simulink model "Cosim"  (R2020b)
settings: Solver=VariableStepAuto  StartTime=0.0  StopTime=15  RelTol=1e-3
values from neighbouring files (symbols this model uses):
  D1_Open = D1_Time + Gripper_Time    (= 4.1)    [Project_Script.m]
  D1_Time = M1_Close + Move_Time    (= 4.05)    [Project_Script.m]
  D2_Open = D2_Time + Gripper_Time    (= 10.2)    [Project_Script.m]
  D2_Time = M2_Close + Move_Time    (= 10.15)    [Project_Script.m]
  D2_Time1 = D1_Open + Move_Time    (= 6.1)    [Project_Script.m]
  D3_Time = M3_Close + Move_Time    (= 16.25)    [Project_Script.m]
  D3_Time1 = D2_Open + Move_Time    (= 12.2)    [Project_Script.m]
  Kb1 = 0.0184    [Project_Script.m]
  Km1 = 0.0184    [Project_Script.m]
  L1 = 0.000231    [Project_Script.m]
  M1_Close = M1_Time + Gripper_Time    (= 2.05)    [Project_Script.m]
  M1_Time = Move_Time    (= 2)    [Project_Script.m]
  M2_Close = M2_Time + Gripper_Time    (= 8.15)    [Project_Script.m]
  M2_Time = D2_Time1 + Move_Time    (= 8.1)    [Project_Script.m]
  M3_Close = M3_Time + Gripper_Time    (= 14.25)    [Project_Script.m]
  M3_Time = D3_Time1 + Move_Time    (= 14.2)    [Project_Script.m]
  Motor1_D1 = 0    [Project_Script.m]
  Motor1_D2 = -(360-345.73)-M1    (= -51.7)    [Project_Script.m]
  Motor1_D3 = -(360-330.2)-M1    (= -67.23)    [Project_Script.m]
  Motor1_M1 = 73.97-M1    (= 36.54)    [Project_Script.m]
  Motor1_M2 = 40.54-M1    (= 3.11)    [Project_Script.m]
  Motor1_M3 = 30.31-M1    (= -7.12)    [Project_Script.m]
  Motor2_D1 = 0    [Project_Script.m]
  Motor2_D2 = -(46.53-M2)    (= 17.05)    [Project_Script.m]
  Motor2_D3 = -(63.66-M2)    (= -0.08)    [Project_Script.m]
  Motor2_M1 = -(124.27-M2)    (= -60.69)    [Project_Script.m]
  Motor2_M2 = -(108.21-M2)    (= -44.63)    [Project_Script.m]
  Motor2_M3 = -(124.23-M2)    (= -60.65)    [Project_Script.m]
  Motor3_D1 = 0    [Project_Script.m]
  Motor3_D2 = 150.8-M3    (= 34.65)    [Project_Script.m]
  Motor3_D3 = 183.46-M3    (= 67.31)    [Project_Script.m]
  Motor3_M1 = 140.3-M3    (= 24.15)    [Project_Script.m]
  Motor3_M2 = 157.67-M3    (= 41.52)    [Project_Script.m]
  Motor3_M3 = 183.92-M3    (= 67.77)    [Project_Script.m]
  Motor4_Closed = -90    [Project_Script.m]
  Motor4_Open = 0    [Project_Script.m]
  R1 = 3.69    [Project_Script.m]
  res = 2*pi/1024    (= 0.00613592315154)    [Project_Script.m]
  Sample_Time = 10000    [Project_Script.m]
libraries: cstblocks x8
settings Model: Creator=deniz  LastModifiedBy=tnurs

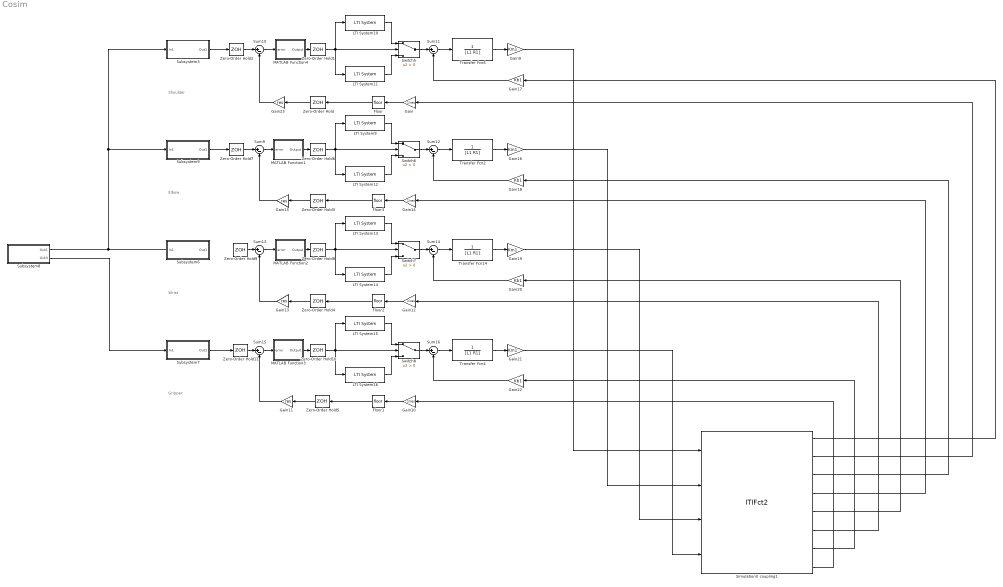
== system Cosim ==
  note: Gripper
  note: Shoulder
  note: Elbow
  note: Wrist
  Floor{,1..3} (4 alike) : Rounding
  Gain{,10,12,14} (4 alike) : Gain  Gain=1/res
  Gain{11,13,15,23} (4 alike) : Gain  Gain=res
  Gain{9,16,19,21} (4 alike) : Gain  Gain=Km1
  Gain{17..18,20,22} (4 alike) : Gain  Gain=Kb1
  LTI System{9..10,13,15} (4 alike) : cstblocks/LTI System  sys=Amp_tf_CW  IC=[]
  LTI System{11..12,14,16} (4 alike) : cstblocks/LTI System  sys=Amp_tf_CCW  IC=[]
  MATLAB Function1 : MATLAB Function  TreatAsAtomicUnit=on
  MATLAB Function2 : MATLAB Function  TreatAsAtomicUnit=on
  MATLAB Function3 : MATLAB Function  TreatAsAtomicUnit=on
  MATLAB Function4 : MATLAB Function  TreatAsAtomicUnit=on
  SimulationX coupling1 : S-Function  FunctionName=ITIFct2  Parameters=ip, port, ts, nIn, nOut  SFunctionDeploymentMode=off  EnableBusSupport=off  mask{ip='localhost', port=4097, ts=0.001, nIn=4, nOut=8}
      mask prompts: ip "Address: ip"; port "Port Number: port [-]"; ts "Communication Step Size: ts [s]"; nIn "Input Vector Dimension (to SimulationX): nIn [-]"; nOut "Output Vector Dimension (from SimulationX): nOut [-]"
      mask help: Coupling Element
  Subsystem3 : Subsystem
  Subsystem6 : Subsystem
  Subsystem7 : Subsystem
  Subsystem8 : Subsystem
  Subsystem9 : Subsystem
  Sum{9..16} (8 alike) : Sum  Inputs=|+-
  Switch{5..8} (4 alike) : Switch  Criteria=u2 > Threshold
  Transfer Fcn{2,4,6,14} (4 alike) : TransferFcn  Denominator=[L1 R1]
  Zero-Order Hold{,1..11} (12 alike) : ZeroOrderHold  SampleTime=1/Sample_Time
  wires:
  MATLAB Function3/1(Output) -> Zero-Order Hold10/1
  Sum13/1 -> MATLAB Function2/1(error)
  Zero-Order Hold1/1 -> Switch5/2, LTI System11/1, LTI System10/1
  Zero-Order Hold3/1 -> Gain15/1
  Zero-Order Hold11/1 -> Sum15/1
  Zero-Order Hold6/1 -> Switch6/2, LTI System12/1, LTI System9/1
  MATLAB Function2/1(Output) -> Zero-Order Hold8/1
  Zero-Order Hold8/1 -> Switch7/2, LTI System13/1, LTI System14/1
  Zero-Order Hold2/1 -> Sum10/1
  Zero-Order Hold5/1 -> Gain11/1
  Sum10/1 -> MATLAB Function4/1(error)
  MATLAB Function4/1(Output) -> Zero-Order Hold1/1
  Floor2/1 -> Zero-Order Hold4/1
  Sum15/1 -> MATLAB Function3/1(error)
  Floor3/1 -> Zero-Order Hold3/1
  Zero-Order Hold9/1 -> Sum13/1
  Sum9/1 -> MATLAB Function1/1(error)
  MATLAB Function1/1(Output) -> Zero-Order Hold6/1
  Gain12/1 -> Floor2/1
  Gain23/1 -> Sum10/2
  Zero-Order Hold10/1 -> Switch8/2, LTI System16/1, LTI System15/1
  Gain/1 -> Floor/1
  Zero-Order Hold/1 -> Gain23/1
  Gain14/1 -> Floor3/1
  Switch5/1 -> Sum11/1
  Floor/1 -> Zero-Order Hold/1
  Transfer Fcn6/1 -> Gain9/1
  Zero-Order Hold7/1 -> Sum9/1
  Gain17/1 -> Sum11/2
  LTI System11/1 -> Switch5/3
  Gain15/1 -> Sum9/2
  Gain11/1 -> Sum15/2
  Subsystem8/1(Out1) -> Subsystem9/1(In1), Subsystem3/1(In1)
  LTI System13/1 -> Switch7/1
  Gain13/1 -> Sum13/2
  Zero-Order Hold4/1 -> Gain13/1
  Transfer Fcn2/1 -> Gain16/1
  Sum11/1 -> Transfer Fcn6/1
  Floor1/1 -> Zero-Order Hold5/1
  LTI System9/1 -> Switch6/1
  Gain22/1 -> Sum16/2
  LTI System10/1 -> Switch5/1
  LTI System16/1 -> Switch8/3
  Sum16/1 -> Transfer Fcn4/1
  Gain18/1 -> Sum12/2
  Gain10/1 -> Floor1/1
  Transfer Fcn4/1 -> Gain21/1
  LTI System15/1 -> Switch8/1
  Sum14/1 -> Transfer Fcn14/1
  Sum12/1 -> Transfer Fcn2/1
  Switch7/1 -> Sum14/1
  Switch8/1 -> Sum16/1
  Switch6/1 -> Sum12/1
  LTI System14/1 -> Switch7/3
  Transfer Fcn14/1 -> Gain19/1
  LTI System12/1 -> Switch6/3
  Subsystem8/2(Out3) -> Subsystem7/1(In1)
  Gain20/1 -> Sum14/2
  Subsystem7/1(Out1) -> Zero-Order Hold11/1
  SimulationX coupling1/8 -> Gain10/1
  SimulationX coupling1/7 -> Gain22/1
  SimulationX coupling1/6 -> Gain12/1
  SimulationX coupling1/5 -> Gain20/1
  SimulationX coupling1/4 -> Gain14/1
  SimulationX coupling1/3 -> Gain18/1
  SimulationX coupling1/2 -> Gain/1
  SimulationX coupling1/1 -> Gain17/1
  Gain16/1 -> SimulationX coupling1/2
  Gain19/1 -> SimulationX coupling1/3
  Gain21/1 -> SimulationX coupling1/4
  Gain9/1 -> SimulationX coupling1/1
  Subsystem3/1(Out1) -> Zero-Order Hold2/1
  ? -> Zero-Order Hold9/1
  Subsystem9/1(Out1) -> Zero-Order Hold7/1

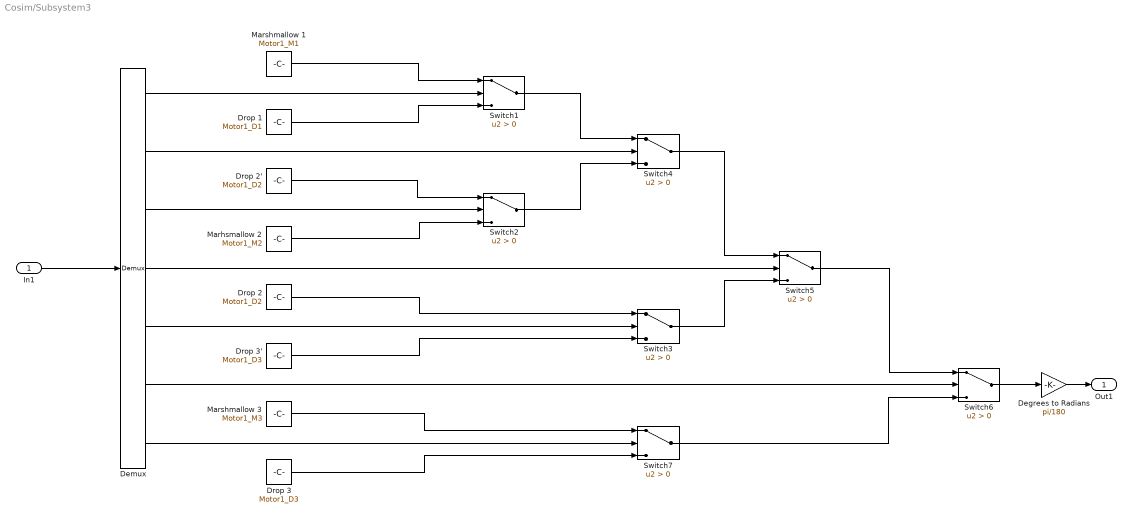
== system Cosim/Subsystem3 ==
  In1 : Inport
  Degrees to Radians : Gain  Gain=pi/180
  Demux : Demux  Outputs=7
  Drop 1 : Constant  Value=Motor1_D1
  Drop 2 : Constant  Value=Motor1_D2
  Drop 2' : Constant  Value=Motor1_D2  VectorParams1D=off
  Drop 3 : Constant  Value=Motor1_D3
  Drop 3' : Constant  Value=Motor1_D3
  Marhsmallow 2 : Constant  Value=Motor1_M2
  Marshmallow 1 : Constant  Value=Motor1_M1
  Marshmallow 3 : Constant  Value=Motor1_M3
  Switch{1..7} (7 alike) : Switch  Criteria=u2 > Threshold
  Out1 : Outport
  wires:
  Marshmallow 1/1 -> Switch1/1
  Drop 1/1 -> Switch1/3
  Drop 2'/1 -> Switch2/1
  Drop 2/1 -> Switch3/1
  Demux/3 -> Switch2/2
  Switch1/1 -> Switch4/1
  Switch2/1 -> Switch4/3
  Switch4/1 -> Switch5/1
  Switch3/1 -> Switch5/3
  Demux/2 -> Switch4/2
  Demux/4 -> Switch5/2
  Drop 3'/1 -> Switch3/3
  Demux/1 -> Switch1/2
  Degrees to Radians/1 -> Out1/1
  Demux/5 -> Switch3/2
  In1/1 -> Demux/1
  Marhsmallow 2/1 -> Switch2/3
  Demux/6 -> Switch6/2
  Switch5/1 -> Switch6/1
  Marshmallow 3/1 -> Switch7/1
  Drop 3/1 -> Switch7/3
  Switch7/1 -> Switch6/3
  Demux/7 -> Switch7/2
  Switch6/1 -> Degrees to Radians/1

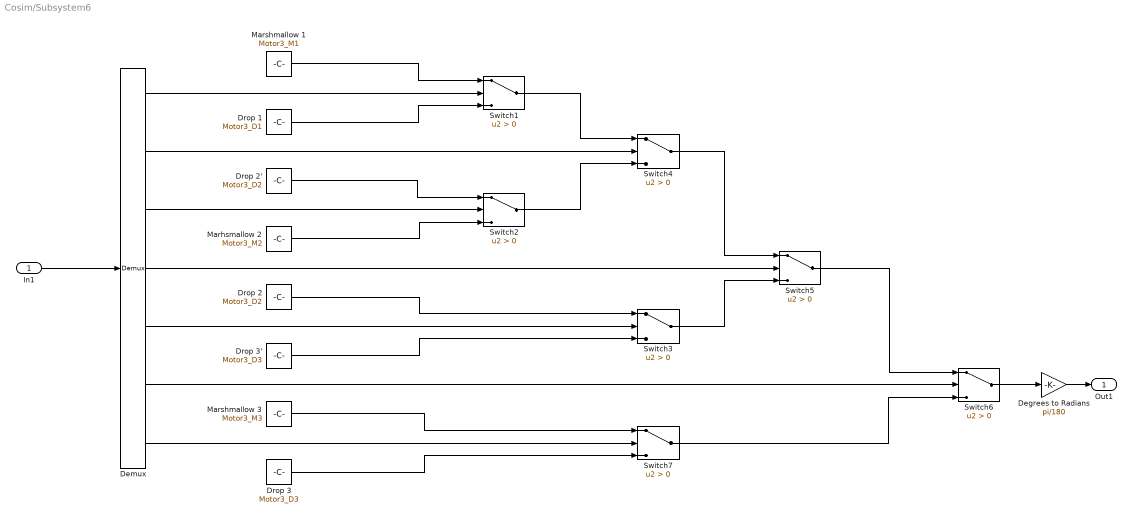
== system Cosim/Subsystem6 ==
  In1 : Inport
  Degrees to Radians : Gain  Gain=pi/180
  Demux : Demux  Outputs=7
  Drop 1 : Constant  Value=Motor3_D1
  Drop 2 : Constant  Value=Motor3_D2
  Drop 2' : Constant  Value=Motor3_D2  VectorParams1D=off
  Drop 3 : Constant  Value=Motor3_D3
  Drop 3' : Constant  Value=Motor3_D3
  Marhsmallow 2 : Constant  Value=Motor3_M2
  Marshmallow 1 : Constant  Value=Motor3_M1
  Marshmallow 3 : Constant  Value=Motor3_M3
  Switch{1..7} (7 alike) : Switch  Criteria=u2 > Threshold
  Out1 : Outport
  wires:
  Drop 3'/1 -> Switch3/3
  Demux/1 -> Switch1/2
  Demux/2 -> Switch4/2
  Marhsmallow 2/1 -> Switch2/3
  In1/1 -> Demux/1
  Drop 1/1 -> Switch1/3
  Switch5/1 -> Switch6/1
  Drop 2'/1 -> Switch2/1
  Switch3/1 -> Switch5/3
  Degrees to Radians/1 -> Out1/1
  Switch4/1 -> Switch5/1
  Switch2/1 -> Switch4/3
  Drop 2/1 -> Switch3/1
  Demux/6 -> Switch6/2
  Switch1/1 -> Switch4/1
  Marshmallow 1/1 -> Switch1/1
  Demux/4 -> Switch5/2
  Demux/7 -> Switch7/2
  Marshmallow 3/1 -> Switch7/1
  Switch6/1 -> Degrees to Radians/1
  Demux/3 -> Switch2/2
  Switch7/1 -> Switch6/3
  Drop 3/1 -> Switch7/3
  Demux/5 -> Switch3/2

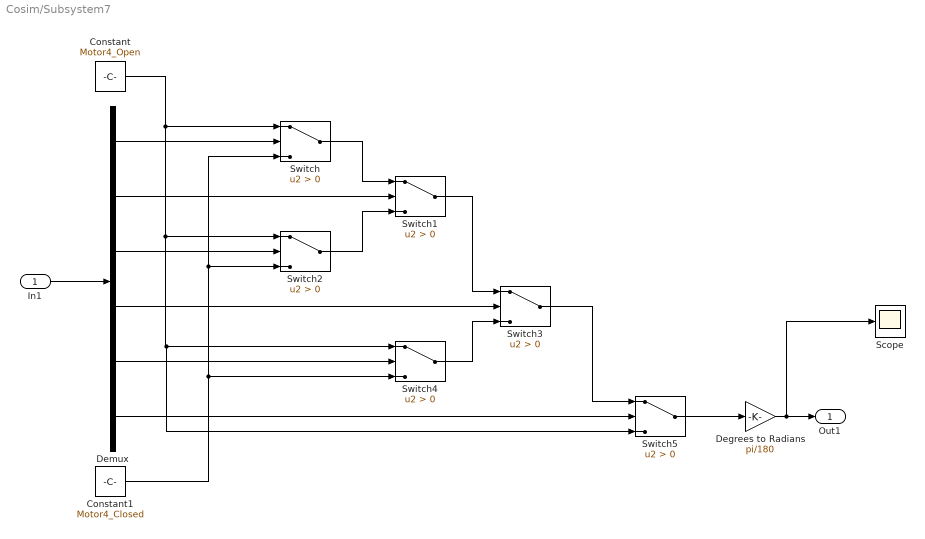
== system Cosim/Subsystem7 ==
  In1 : Inport
  Constant : Constant  Value=Motor4_Open
  Constant1 : Constant  Value=Motor4_Closed
  Degrees to Radians : Gain  Gain=pi/180
  Demux : Demux  Outputs=6
  Scope : Scope
  Switch{,1..5} (6 alike) : Switch  Criteria=u2 > Threshold
  Out1 : Outport
  wires:
  Switch5/1 -> Degrees to Radians/1
  In1/1 -> Demux/1
  Degrees to Radians/1 -> Scope/1, Out1/1
  Constant/1 -> Switch5/3, Switch4/1, Switch2/1, Switch/1
  Demux/1 -> Switch/2
  Constant1/1 -> Switch4/3, Switch2/3, Switch/3
  Demux/2 -> Switch1/2
  Switch/1 -> Switch1/1
  Switch2/1 -> Switch1/3
  Demux/3 -> Switch2/2
  Demux/4 -> Switch3/2
  Switch1/1 -> Switch3/1
  Switch4/1 -> Switch3/3
  Demux/5 -> Switch4/2
  Demux/6 -> Switch5/2
  Switch3/1 -> Switch5/1

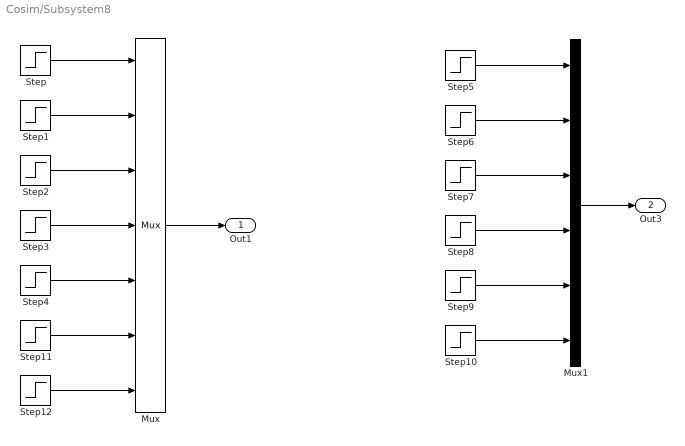
== system Cosim/Subsystem8 ==
  Mux : Mux  Inputs=7
  Mux1 : Mux  Inputs=6
  Step : Step  Time=M1_Close  Before=1  After=0  SampleTime=0
  Step1 : Step  Time=D1_Open  Before=1  After=0  SampleTime=0
  Step10 : Step  Time=D3_Time  Before=1  After=0  SampleTime=0
  Step11 : Step  Time=D3_Time1  Before=1  After=0  SampleTime=0
  Step12 : Step  Time=M3_Close  Before=1  After=0  SampleTime=0
  Step2 : Step  Time=D2_Time1  Before=1  After=0  SampleTime=0
  Step3 : Step  Time=M2_Close  Before=1  After=0  SampleTime=0
  Step4 : Step  Time=D2_Open  Before=1  After=0  SampleTime=0
  Step5 : Step  Time=M1_Time  Before=1  After=0  SampleTime=0
  Step6 : Step  Time=D1_Time  Before=1  After=0  SampleTime=0
  Step7 : Step  Time=M2_Time  Before=1  After=0  SampleTime=0
  Step8 : Step  Time=D2_Time  Before=1  After=0  SampleTime=0
  Step9 : Step  Time=M3_Time  Before=1  After=0  SampleTime=0
  Out1 : Outport
  Out3 : Outport  Port=2
  wires:
  Mux/1 -> Out1/1
  Step4/1 -> Mux/5
  Step3/1 -> Mux/4
  Step2/1 -> Mux/3
  Step1/1 -> Mux/2
  Step/1 -> Mux/1
  Step8/1 -> Mux1/4
  Step6/1 -> Mux1/2
  Step9/1 -> Mux1/5
  Mux1/1 -> Out3/1
  Step7/1 -> Mux1/3
  Step5/1 -> Mux1/1
  Step10/1 -> Mux1/6
  Step11/1 -> Mux/6
  Step12/1 -> Mux/7

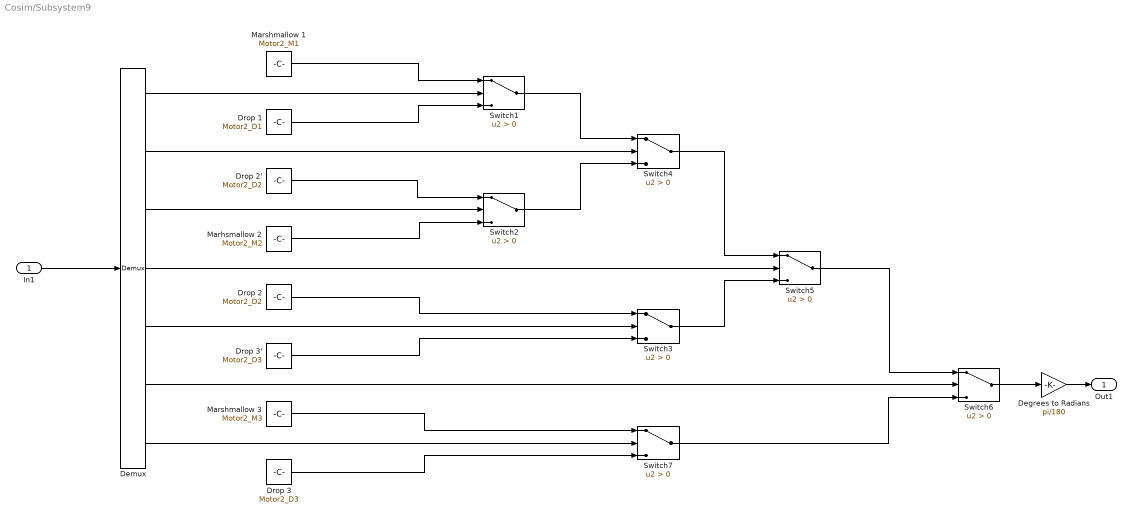
== system Cosim/Subsystem9 ==
  In1 : Inport
  Degrees to Radians : Gain  Gain=pi/180
  Demux : Demux  Outputs=7
  Drop 1 : Constant  Value=Motor2_D1
  Drop 2 : Constant  Value=Motor2_D2
  Drop 2' : Constant  Value=Motor2_D2  VectorParams1D=off
  Drop 3 : Constant  Value=Motor2_D3
  Drop 3' : Constant  Value=Motor2_D3
  Marhsmallow 2 : Constant  Value=Motor2_M2
  Marshmallow 1 : Constant  Value=Motor2_M1
  Marshmallow 3 : Constant  Value=Motor2_M3
  Switch{1..7} (7 alike) : Switch  Criteria=u2 > Threshold
  Out1 : Outport
  wires:
  Drop 3'/1 -> Switch3/3
  Demux/1 -> Switch1/2
  Demux/2 -> Switch4/2
  Marhsmallow 2/1 -> Switch2/3
  In1/1 -> Demux/1
  Drop 1/1 -> Switch1/3
  Switch5/1 -> Switch6/1
  Drop 2'/1 -> Switch2/1
  Switch3/1 -> Switch5/3
  Degrees to Radians/1 -> Out1/1
  Switch4/1 -> Switch5/1
  Switch2/1 -> Switch4/3
  Drop 2/1 -> Switch3/1
  Demux/6 -> Switch6/2
  Switch1/1 -> Switch4/1
  Marshmallow 1/1 -> Switch1/1
  Demux/4 -> Switch5/2
  Demux/7 -> Switch7/2
  Marshmallow 3/1 -> Switch7/1
  Switch6/1 -> Degrees to Radians/1
  Demux/3 -> Switch2/2
  Switch7/1 -> Switch6/3
  Drop 3/1 -> Switch7/3
  Demux/5 -> Switch3/2

== matlab function Cosim/MATLAB Function2 ==
  settings: sampleTime=1/10000
  data: error input; Output output
function Output = PID(error)

persistent ept              %holds the exponentials
persistent results          %holds reccorded derivatives
persistent previous_error   %holds input from last execution for derivative calc
persistent integral         %holds the total integral
CF = 10000;                 %ISR frequency
delta_t = 1/CF;             %Will change according to CF, sampling time
size = 8;                   %can change between 5-10
n = 4;                      %Decaying until n*tau, can be 4 or 5
pole = n*CF/size;
P_gain = 0.2616;
D_gain = 0.0432;
%I_gain = 13.390;
I_gain = 0.01;

%initialize vectors and variables
if isempty(results)
    results = zeros(1,size);
    ept = zeros(1,size);
    sum = 0;
    integral = 0;
    previous_error = 0;
    
    %calculate scale factor for derivative
    for i = 1:size
        sum = sum + pole*exp(-pole*i*delta_t);
    end
    Scale_Factor = 1/(sum);
    
    %properly create ept
    for i = 1:size
        ept(i) = Scale_Factor*pole*exp(-pole*i*delta_t);
    end
end

%Calculating the D(Derivative) of PID
results(2:size)=results(1:size-1);
results(1)=(error - previous_error)/delta_t;
previous_error = error;
derivative = dot(results,ept);

%Calculating the I(Integral) of PID
integral = integral + (error + previous_error)/2*delta_t;

%Calculating the P(Proportional) of PID
proportional = error*P_gain;

Output = proportional + I_gain*integral + D_gain*derivative;

== matlab function Cosim/MATLAB Function3 ==
  settings: sampleTime=1/10000
  data: error input; Output output
function Output = PID(error)

persistent ept              %holds the exponentials
persistent results          %holds reccorded derivatives
persistent previous_error   %holds input from last execution for derivative calc
persistent integral         %holds the total integral
CF = 10000;                 %ISR frequency
delta_t = 1/CF;             %Will change according to CF, sampling time
size = 8;                   %can change between 5-10
n = 4;                      %Decaying until n*tau, can be 4 or 5
pole = n*CF/size;
P_gain = 0.2616;
D_gain = 0.0432;
I_gain = 0.01;
%I_gain = 13.390;

%initialize vectors and variables
if isempty(results)
    results = zeros(1,size);
    ept = zeros(1,size);
    sum = 0;
    integral = 0;
    previous_error = 0;
    
    %calculate scale factor for derivative
    for i = 1:size
        sum = sum + pole*exp(-pole*i*delta_t);
    end
    Scale_Factor = 1/(sum);
    
    %properly create ept
    for i = 1:size
        ept(i) = Scale_Factor*pole*exp(-pole*i*delta_t);
    end
end

%Calculating the D(Derivative) of PID
results(2:size)=results(1:size-1);
results(1)=(error - previous_error)/delta_t;
previous_error = error;
derivative = dot(results,ept);

%Calculating the I(Integral) of PID
integral = integral + (error + previous_error)/2*delta_t;

%Calculating the P(Proportional) of PID
proportional = error*P_gain;

%Output = proportional;
Output = proportional + I_gain*integral + D_gain*derivative;

== matlab function Cosim/MATLAB Function4 ==
  settings: sampleTime=1/10000
  data: error input; Output output
function Output = PID(error)

persistent ept              %holds the exponentials
persistent results          %holds reccorded derivatives
persistent previous_error   %holds input from last execution for derivative calc
persistent integral         %holds the total integral
CF = 10000;                 %ISR frequency
delta_t = 1/CF;             %Will change according to CF, sampling time
size = 8;                   %can change between 5-10
n = 4;                      %Decaying until n*tau, can be 4 or 5
pole = n*CF/size;
P_gain = 0.2616;
%P_gain = 0.2616;
D_gain = 0.9;
%D_gain = 0.0432;
%I_gain = 13.390;
I_gain = 0.01;

%initialize vectors and variables
if isempty(results)
    results = zeros(1,size);
    ept = zeros(1,size);
    sum = 0;
    integral = 0;
    previous_error = 0;
    
    %calculate scale factor for derivative
    for i = 1:size
        sum = sum + pole*exp(-pole*i*delta_t);
    end
    Scale_Factor = 1/(sum);
    
    %properly create ept
    for i = 1:size
        ept(i) = Scale_Factor*pole*exp(-pole*i*delta_t);
    end
end

%Calculating the D(Derivative) of PID
results(2:size)=results(1:size-1);
results(1)=(error - previous_error)/delta_t;
previous_error = error;
derivative = dot(results,ept);

%Calculating the I(Integral) of PID
integral = integral + (error + previous_error)/2*delta_t;

%Calculating the P(Proportional) of PID
proportional = error*P_gain;

Output = proportional + I_gain*integral + D_gain*derivative;

== matlab function Cosim/MATLAB Function1 ==
  settings: sampleTime=1/10000
  data: error input; Output output
function Output = PID(error)

persistent ept              %holds the exponentials
persistent results          %holds reccorded derivatives
persistent previous_error   %holds input from last execution for derivative calc
persistent integral         %holds the total integral
CF = 10000;                 %ISR frequency
delta_t = 1/CF;             %Will change according to CF, sampling time
size = 8;                   %can change between 5-10
n = 4;                      %Decaying until n*tau, can be 4 or 5
pole = n*CF/size;
P_gain = 0.15;
%P_gain = 0.2616;
%D_gain = 0.0432;
D_gain = 1.5;
%I_gain = 13.390;
I_gain = 0.05;

%initialize vectors and variables
if isempty(results)
    results = zeros(1,size);
    ept = zeros(1,size);
    sum = 0;
    integral = 0;
    previous_error = 0;
    
    %calculate scale factor for derivative
    for i = 1:size
        sum = sum + pole*exp(-pole*i*delta_t);
    end
    Scale_Factor = 1/(sum);
    
    %properly create ept
    for i = 1:size
        ept(i) = Scale_Factor*pole*exp(-pole*i*delta_t);
    end
end

%Calculating the D(Derivative) of PID
results(2:size)=results(1:size-1);
results(1)=(error - previous_error)/delta_t;
previous_error = error;
derivative = dot(results,ept);

%Calculating the I(Integral) of PID
integral = integral + (error + previous_error)/2*delta_t;

%Calculating the P(Proportional) of PID
proportional = error*P_gain;

Output = proportional + I_gain*integral + D_gain*derivative;
